simulink model "PIDTest2"  (R2013b)
settings: Solver=ode45  StartTime=0.0  StopTime=20  RelTol=1e-3
settings Model: Creator=Deepak  LastModifiedBy=Deepak

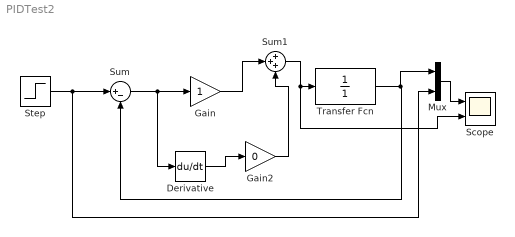
== system PIDTest2 ==
  Derivative : Derivative
  Gain : Gain
  Gain2 : Gain  Gain=0
  Mux : Mux  Inputs=2
  Scope : Scope  NumInputPorts=2
      settings: TimeRange=20  YMin=-5~-5  YMax=5~5
  Step : Step  SampleTime=0
  Sum : Sum  Inputs=|+-
  Sum1 : Sum  Inputs=+++
  Transfer Fcn : TransferFcn  Denominator=[1]
  wires:
  Transfer Fcn/1 -> Mux/1, Sum/2
  Step/1 -> Mux/2, Sum/1
  Sum/1 -> Derivative/1, Gain/1
  Mux/1 -> Scope/1
  Gain/1 -> Sum1/2
  Sum1/1 -> Scope/2, Transfer Fcn/1
  Derivative/1 -> Gain2/1
  Gain2/1 -> Sum1/3
